simulink model "sampleModel20"  (R2021a)
settings: Solver=VariableStepAuto  StartTime=0.0  StopTime=10.0  RelTol=1e-3
undefined symbols (not defined in the file): DiscIntNeverNeededParam, magnitude, Newton, Raphson
libraries: simulink x274, pid_lib x17
(part 14 of 16)

== system sampleModel20/cfblk90/cfblk9/cfblk9/cfblk5 ==
  cfblk1 : Inport
  cfblk8 : Inport  Port=2
  cfblk10 : Delay  SampleTime=1
  cfblk3 : DiscreteFir  SampleTime=1
  cfblk4 : Sin  TimeSource=Use external signal  SampleTime=0
  cfblk5 : Sum  Inputs=+-
  cfblk6 : ComplexToRealImag
  cfblk7 : MinMax  Inputs=2
  cfblk2 : Outport
  cfblk9 : Outport  Port=2
  wires:
  cfblk8/1 -> cfblk2/1
  cfblk1/1 -> cfblk5/1, cfblk7/2
  cfblk3/1 -> cfblk4/1
  cfblk7/1 -> cfblk6/1
  cfblk5/1 -> cfblk3/1
  cfblk4/1 -> cfblk9/1
  cfblk6/1 -> cfblk5/2
  cfblk6/2 -> cfblk10/1
  cfblk10/1 -> cfblk7/1

== system sampleModel20/cfblk90/cfblk9/cfblk9/cfblk6 ==
  cfblk1 : Inport
  cfblk5 : Inport  Port=2
  cfblk6 : Inport  Port=3
  cfblk7 : Inport  Port=4
  cfblk8 : Inport  Port=5
  cfblk9 : Inport  Port=6
  cfblk10 : Inport  Port=7
  cfblk3 : Reshape
  cfblk4 : Product
  cfblk2 : Outport
  wires:
  cfblk10/1 -> cfblk2/1
  cfblk5/1 -> cfblk4/1
  cfblk1/1 -> cfblk4/2
  cfblk4/1 -> cfblk3/1

== system sampleModel20/cfblk90/cfblk9/cfblk9/cfblk7 ==
  cfblk1 : Inport
  cfblk7 : Inport  Port=2
  cfblk3 : simulink/Math Operations/Slider Gain  gain=1  low=0  high=2
  cfblk4 : Sum  Inputs=+-
  cfblk5 : Product
  cfblk6 : Bias  Bias=[368152443.694758]
  cfblk8 : Delay  SampleTime=1
  cfblk2 : Outport
  wires:
  cfblk3/1 -> cfblk2/1
  cfblk7/1 -> cfblk4/2
  cfblk1/1 -> cfblk3/1
  cfblk4/1 -> cfblk6/1, cfblk5/2
  cfblk6/1 -> cfblk5/1
  cfblk5/1 -> cfblk8/1
  cfblk8/1 -> cfblk4/1

== system sampleModel20/cfblk90/cfblk9/cfblk9/cfblk8 ==
  cfblk1 : Inport
  cfblk6 : Inport  Port=2
  cfblk7 : Inport  Port=3
  cfblk8 : Inport  Port=4
  cfblk9 : Inport  Port=5
  cfblk10 : Inport  Port=6
  cfblk3 : DiscreteTransferFcn  SampleTime=1
  cfblk4 : Product  Inputs=*
  cfblk5 : Reshape
  cfblk2 : Outport
  cfblk11 : Outport  Port=2
  wires:
  cfblk5/1 -> cfblk11/1
  cfblk9/1 -> cfblk5/1
  cfblk10/1 -> cfblk3/1
  cfblk8/1 -> cfblk2/1
  cfblk6/1 -> cfblk4/1

== system sampleModel20/cfblk90/cfblk9/cfblk9/cfblk9 ==
  cfblk1 : Inport
  cfblk10 : Inport  Port=2
  cfblk11 : Inport  Port=3
  cfblk12 : Inport  Port=4
  cfblk13 : Inport  Port=5
  cfblk14 : Inport  Port=6
  cfblk15 : Inport  Port=7
  cfblk17 : Delay  SampleTime=1
  cfblk3 : PermuteDimensions
  cfblk4 : Rounding
  cfblk5 : Product
  cfblk6 : UnaryMinus
  cfblk7 : Signum
  cfblk8 : simulink/Math Operations/Slider Gain  gain=1  low=0  high=2
  cfblk9 : Signum
  cfblk2 : Outport
  cfblk16 : Outport  Port=2
  wires:
  cfblk4/1 -> cfblk3/1
  cfblk7/1 -> cfblk16/1
  cfblk11/1 -> cfblk7/1
  cfblk15/1 -> cfblk6/1
  cfblk10/1 -> cfblk2/1
  cfblk6/1 -> cfblk4/1
  cfblk5/1 -> cfblk8/1
  cfblk1/1 -> cfblk9/1
  cfblk9/1 -> cfblk5/2
  cfblk8/1 -> cfblk17/1
  cfblk17/1 -> cfblk5/1

== system sampleModel20/cfblk91/cfblk5/cfblk10/cfblk10 ==
  cfblk1 : Inport
  cfblk5 : Inport  Port=2
  cfblk6 : Inport  Port=3
  cfblk7 : Inport  Port=4
  cfblk8 : Inport  Port=5
  cfblk9 : Inport  Port=6
  cfblk3 : Sum  Inputs=+-
  cfblk4 : Sum  Inputs=|++
  cfblk2 : Outport
  cfblk10 : Outport  Port=2
  wires:
  cfblk4/1 -> cfblk3/1
  cfblk8/1 -> cfblk2/1
  cfblk7/1 -> cfblk3/2
  cfblk6/1 -> cfblk10/1
  cfblk5/1 -> cfblk4/1
  cfblk1/1 -> cfblk4/2

== system sampleModel20/cfblk91/cfblk5/cfblk10/cfblk11 ==
  cfblk1 : Inport
  cfblk8 : Inport  Port=2
  cfblk9 : Inport  Port=3
  cfblk10 : Inport  Port=4
  cfblk11 : Inport  Port=5
  cfblk12 : Inport  Port=6
  cfblk13 : Inport  Port=7
  cfblk3 : Sqrt  SaturateOnIntegerOverflow=on
  cfblk4 : Sin  TimeSource=Use external signal  SampleTime=0
  cfblk5 : MinMax  Function=max  Inputs=3
  cfblk6 : Squeeze
  cfblk7 : Math  Operator=log10  SaturateOnIntegerOverflow=on
  cfblk2 : Outport
  cfblk14 : Outport  Port=2
  cfblk15 : Outport  Port=3
  wires:
  cfblk11/1 -> cfblk6/1
  cfblk5/1 -> cfblk4/1
  cfblk7/1 -> cfblk15/1
  cfblk1/1 -> cfblk14/1
  cfblk9/1 -> cfblk3/1
  cfblk6/1 -> cfblk2/1
  cfblk8/1 -> cfblk5/1
  cfblk3/1 -> cfblk5/2
  cfblk12/1 -> cfblk7/1
  cfblk13/1 -> cfblk5/3

== system sampleModel20/cfblk91/cfblk5/cfblk10/cfblk12 ==
  cfblk1 : Inport
  cfblk7 : Inport  Port=2
  cfblk8 : Inport  Port=3
  cfblk9 : Inport  Port=4
  cfblk10 : Inport  Port=5
  cfblk11 : Inport  Port=6
  cfblk3 : Sqrt  SaturateOnIntegerOverflow=on
  cfblk4 : Sin  TimeSource=Use external signal  SampleTime=0
  cfblk5 : DotProduct  InputSameDT=on  OutDataTypeStr=Inherit: Inherit via internal rule
  cfblk6 : Polyval  Coefs=[ +2.081618890e-019, -1.441693666e-014, +4.719686976e-010, -8.536869453e-006, +1.621573104e-001, -8.087801117e+001 ]
  cfblk2 : Outport
  cfblk12 : Outport  Port=2
  wires:
  cfblk9/1 -> cfblk5/1
  cfblk11/1 -> cfblk6/1
  cfblk1/1 -> cfblk2/1
  cfblk8/1 -> cfblk4/1
  cfblk5/1 -> cfblk12/1
  cfblk6/1 -> cfblk5/2
  cfblk10/1 -> cfblk3/1

== system sampleModel20/cfblk91/cfblk5/cfblk10/cfblk13 ==
  cfblk1 : Inport
  cfblk5 : Inport  Port=2
  cfblk6 : Inport  Port=3
  cfblk7 : Inport  Port=4
  cfblk3 : Reshape
  cfblk4 : Sin  TimeSource=Use external signal  SampleTime=0
  cfblk2 : Outport
  cfblk8 : Outport  Port=2
  cfblk9 : Outport  Port=3
  wires:
  cfblk6/1 -> cfblk2/1
  cfblk4/1 -> cfblk9/1
  cfblk5/1 -> cfblk4/1
  cfblk1/1 -> cfblk8/1
  cfblk7/1 -> cfblk3/1

== system sampleModel20/cfblk91/cfblk5/cfblk4/cfblk4 ==
  cfblk1 : Inport
  cfblk13 : Inport  Port=2
  cfblk14 : Inport  Port=3
  cfblk10 : Sum  Inputs=|++
  cfblk11 : Polyval  Coefs=[ +2.081618890e-019, -1.441693666e-014, +4.719686976e-010, -8.536869453e-006, +1.621573104e-001, -8.087801117e+001 ]
  cfblk12 : Assignment  DiagnosticForDimensions=Warning  IndexOptions=Index vector (dialog)  Indices=1  OutputSizes=1
  cfblk15 : Delay  SampleTime=1
  cfblk16 : Delay  SampleTime=1
  cfblk3 : Rounding
  cfblk4 : ComplexToRealImag
  cfblk5 : Abs
  cfblk6 : Sum  Inputs=|++
  cfblk7 : ComplexToMagnitudeAngle
  cfblk8 : simulink/Math Operations/MinMax Running Resettable  Function=min  vinit=0.0
  cfblk9 : Product  Inputs=**
  cfblk2 : Outport
  wires:
  cfblk14/1 -> cfblk12/1
  cfblk1/1 -> cfblk4/1, cfblk5/1
  cfblk4/1 -> cfblk2/1
  cfblk13/1 -> cfblk10/1
  cfblk6/1 -> cfblk7/1
  cfblk9/1 -> cfblk3/1
  cfblk11/1 -> cfblk6/2
  cfblk12/1 -> cfblk9/1
  cfblk7/2 -> cfblk8/2
  cfblk8/1 -> cfblk12/2
  cfblk10/1 -> cfblk9/2
  cfblk5/1 -> cfblk10/2
  cfblk4/2 -> cfblk11/1
  cfblk7/1 -> cfblk15/1
  cfblk15/1 -> cfblk6/1
  cfblk3/1 -> cfblk16/1
  cfblk16/1 -> cfblk8/1

== system sampleModel20/cfblk91/cfblk5/cfblk4/cfblk5 ==
  cfblk1 : Inport
  cfblk7 : Inport  Port=2
  cfblk8 : Inport  Port=3
  cfblk9 : Inport  Port=4
  cfblk12 : Delay  SampleTime=1
  cfblk3 : ComplexToMagnitudeAngle
  cfblk4 : PermuteDimensions
  cfblk5 : Sin  TimeSource=Use external signal  SampleTime=0
  cfblk6 : Product  Inputs=**
  cfblk2 : Outport
  cfblk10 : Outport  Port=2
  cfblk11 : Outport  Port=3
  wires:
  cfblk3/1 -> cfblk11/1
  cfblk8/1 -> cfblk4/1
  cfblk9/1 -> cfblk10/1
  cfblk1/1 -> cfblk2/1
  cfblk5/1 -> cfblk6/1
  cfblk3/2 -> cfblk5/1
  cfblk7/1 -> cfblk6/2
  cfblk6/1 -> cfblk12/1
  cfblk12/1 -> cfblk3/1

== system sampleModel20/cfblk91/cfblk5/cfblk5/cfblk8 ==
  cfblk1 : Inport
  cfblk10 : Inport  Port=2
  cfblk11 : Inport  Port=3
  cfblk12 : Inport  Port=4
  cfblk13 : Inport  Port=5
  cfblk14 : Inport  Port=6
  cfblk15 : Inport  Port=7
  cfblk16 : Inport  Port=8
  cfblk17 : Inport  Port=9
  cfblk3 : PermuteDimensions
  cfblk4 : Reshape
  cfblk5 : Abs
  cfblk6 : Assignment  DiagnosticForDimensions=Warning  IndexOptions=Index vector (dialog)  Indices=1  OutputSizes=1
  cfblk7 : MinMax  Inputs=2
  cfblk8 : simulink/Math Operations/MinMax Running Resettable  Function=min  vinit=0.0
  cfblk9 : Product  Inputs=**
  cfblk2 : Outport
  wires:
  cfblk6/1 -> cfblk4/1
  cfblk1/1 -> cfblk5/1
  cfblk10/1 -> cfblk6/1
  cfblk17/1 -> cfblk7/1
  cfblk13/1 -> cfblk3/1
  cfblk11/1 -> cfblk9/1
  cfblk14/1 -> cfblk8/1
  cfblk3/1 -> cfblk2/1
  cfblk12/1 -> cfblk9/2
  cfblk8/1 -> cfblk7/2
  cfblk16/1 -> cfblk6/2
  cfblk15/1 -> cfblk8/2

== system sampleModel20/cfblk91/cfblk5/cfblk5/cfblk9 ==
  cfblk1 : Inport
  cfblk5 : Inport  Port=2
  cfblk6 : Inport  Port=3
  cfblk7 : Inport  Port=4
  cfblk3 : Sum  Inputs=+-
  cfblk4 : Sum  Inputs=|++
  cfblk2 : Outport
  wires:
  cfblk3/1 -> cfblk4/1
  cfblk1/1 -> cfblk2/1
  cfblk5/1 -> cfblk4/2
  cfblk7/1 -> cfblk3/1
  cfblk6/1 -> cfblk3/2

== system sampleModel20/cfblk91/cfblk5/cfblk6/cfblk5 ==
  cfblk1 : Inport
  cfblk9 : Inport  Port=2
  cfblk10 : Inport  Port=3
  cfblk11 : Inport  Port=4
  cfblk12 : Inport  Port=5
  cfblk13 : Inport  Port=6
  cfblk14 : Inport  Port=7
  cfblk3 : Sqrt  SaturateOnIntegerOverflow=on
  cfblk4 : Reshape
  cfblk5 : MinMax  Function=max
  cfblk6 : PermuteDimensions
  cfblk7 : ComplexToMagnitudeAngle
  cfblk8 : simulink/Math Operations/Slider Gain  gain=1  low=0  high=2
  cfblk2 : Outport
  wires:
  cfblk8/1 -> cfblk2/1
  cfblk4/1 -> cfblk6/1
  cfblk1/1 -> cfblk5/1
  cfblk12/1 -> cfblk7/1
  cfblk3/1 -> cfblk8/1
  cfblk11/1 -> cfblk4/1
  cfblk9/1 -> cfblk3/1

== system sampleModel20/cfblk91/cfblk5/cfblk7/cfblk5 ==
  cfblk1 : Inport
  cfblk6 : Inport  Port=2
  cfblk7 : Inport  Port=3
  cfblk8 : Inport  Port=4
  cfblk9 : Inport  Port=5
  cfblk10 : Inport  Port=6
  cfblk11 : Inport  Port=7
  cfblk16 : Delay  SampleTime=1
  cfblk3 : Assignment  DiagnosticForDimensions=Warning  IndexOptions=Index vector (dialog)  Indices=1  OutputSizes=1
  cfblk4 : MinMax  Function=max
  cfblk5 : ComplexToMagnitudeAngle
  cfblk2 : Outport
  cfblk12 : Outport  Port=2
  cfblk13 : Outport  Port=3
  cfblk14 : Outport  Port=4
  cfblk15 : Outport  Port=5
  wires:
  cfblk11/1 -> cfblk13/1
  cfblk1/1 -> cfblk2/1
  cfblk3/1 -> cfblk5/1
  cfblk4/1 -> cfblk3/1
  cfblk6/1 -> cfblk4/1
  cfblk9/1 -> cfblk14/1
  cfblk7/1 -> cfblk12/1
  cfblk10/1 -> cfblk15/1
  cfblk5/1 -> cfblk16/1
  cfblk16/1 -> cfblk3/2

== system sampleModel20/cfblk91/cfblk5/cfblk7/cfblk6 ==
  cfblk1 : Inport
  cfblk8 : Inport  Port=2
  cfblk11 : Delay  SampleTime=1
  cfblk3 : Assignment  DiagnosticForDimensions=Warning  IndexOptions=Index vector (dialog)  Indices=1  OutputSizes=1
  cfblk4 : simulink/Math Operations/Slider Gain  gain=1  low=0  high=2
  cfblk5 : Math  Operator=rem  SaturateOnIntegerOverflow=on
  cfblk6 : ComplexToRealImag
  cfblk7 : Constant  Value=[-196577758.764814]  SampleTime=1
  cfblk2 : Outport
  cfblk9 : Outport  Port=2
  cfblk10 : Outport  Port=3
  wires:
  cfblk5/1 -> cfblk4/1
  cfblk8/1 -> cfblk2/1, cfblk3/2
  cfblk1/1 -> cfblk5/1
  cfblk4/1 -> cfblk10/1
  cfblk3/1 -> cfblk6/1
  cfblk7/1 -> cfblk5/2
  cfblk6/1 -> cfblk9/1
  cfblk6/2 -> cfblk11/1
  cfblk11/1 -> cfblk3/1

== system sampleModel20/cfblk91/cfblk5/cfblk7/cfblk7 ==
  cfblk1 : Inport
  cfblk8 : Inport  Port=2
  cfblk9 : Inport  Port=3
  cfblk10 : Inport  Port=4
  cfblk11 : Inport  Port=5
  cfblk12 : Inport  Port=6
  cfblk15 : Delay  SampleTime=1
  cfblk16 : Delay  SampleTime=1
  cfblk3 : Sum  Inputs=|++
  cfblk4 : ComplexToMagnitudeAngle
  cfblk5 : Sum  Inputs=+-
  cfblk6 : Signum
  cfblk7 : Product
  cfblk2 : Outport
  cfblk13 : Outport  Port=2
  cfblk14 : Outport  Port=3
  wires:
  cfblk9/1 -> cfblk5/1
  cfblk12/1 -> cfblk5/2
  cfblk1/1 -> cfblk6/1
  cfblk6/1 -> cfblk2/1
  cfblk11/1 -> cfblk13/1
  cfblk5/1 -> cfblk7/1
  cfblk3/1 -> cfblk4/1
  cfblk8/1 -> cfblk14/1
  cfblk4/2 -> cfblk7/2
  cfblk4/1 -> cfblk15/1
  cfblk15/1 -> cfblk3/2
  cfblk7/1 -> cfblk16/1
  cfblk16/1 -> cfblk3/1

== system sampleModel20/cfblk91/cfblk5/cfblk7/cfblk8 ==
  cfblk1 : Inport
  cfblk5 : Inport  Port=2
  cfblk6 : Inport  Port=3
  cfblk7 : Inport  Port=4
  cfblk3 : Product
  cfblk4 : Bias  Bias=[403133249.538603]
  cfblk2 : Outport
  wires:
  cfblk3/1 -> cfblk4/1
  cfblk4/1 -> cfblk2/1
  cfblk7/1 -> cfblk3/1
  cfblk5/1 -> cfblk3/2

== system sampleModel20/cfblk91/cfblk5/cfblk8/cfblk5 ==
  cfblk1 : Inport
  cfblk6 : Inport  Port=2
  cfblk7 : Inport  Port=3
  cfblk8 : Inport  Port=4
  cfblk9 : Inport  Port=5
  cfblk10 : Inport  Port=6
  cfblk3 : Gain  Gain=[791787314.967177]
  cfblk4 : Gain  Gain=[648519034.471497]
  cfblk5 : Abs
  cfblk2 : Outport
  cfblk11 : Outport  Port=2
  cfblk12 : Outport  Port=3
  cfblk13 : Outport  Port=4
  cfblk14 : Outport  Port=5
  wires:
  cfblk6/1 -> cfblk13/1
  cfblk10/1 -> cfblk2/1
  cfblk3/1 -> cfblk4/1
  cfblk1/1 -> cfblk12/1
  cfblk7/1 -> cfblk14/1
  cfblk8/1 -> cfblk5/1
  cfblk5/1 -> cfblk11/1
  cfblk9/1 -> cfblk3/1

== system sampleModel20/cfblk91/cfblk5/cfblk8/cfblk6 ==
  cfblk1 : Inport
  cfblk4 : Inport  Port=2
  cfblk5 : Inport  Port=3
  cfblk6 : Inport  Port=4
  cfblk7 : Inport  Port=5
  cfblk3 : Sum  Inputs=+
  cfblk2 : Outport
  wires:
  cfblk3/1 -> cfblk2/1
  cfblk1/1 -> cfblk3/1

== system sampleModel20/cfblk91/cfblk5/cfblk8/cfblk7 ==
  cfblk1 : Inport
  cfblk7 : Inport  Port=2
  cfblk8 : Inport  Port=3
  cfblk9 : Inport  Port=4
  cfblk10 : Inport  Port=5
  cfblk11 : Inport  Port=6
  cfblk12 : Inport  Port=7
  cfblk13 : Inport  Port=8
  cfblk15 : Delay  SampleTime=1
  cfblk3 : DiscreteIntegrator  ICPrevOutput=DiscIntNeverNeededParam  ICPrevScaledInput=DiscIntNeverNeededParam
  cfblk4 : DotProduct  InputSameDT=on  OutDataTypeStr=Inherit: Inherit via internal rule
  cfblk5 : Sum  Inputs=+-
  cfblk6 : Assignment  DiagnosticForDimensions=Warning  IndexOptions=Index vector (dialog)  Indices=1  OutputSizes=1
  cfblk2 : Outport
  cfblk14 : Outport  Port=2
  wires:
  cfblk12/1 -> cfblk2/1
  cfblk4/1 -> cfblk6/1
  cfblk8/1 -> cfblk5/1
  cfblk7/1 -> cfblk14/1
  cfblk10/1 -> cfblk5/2
  cfblk1/1 -> cfblk4/2
  cfblk11/1 -> cfblk3/1
  cfblk3/1 -> cfblk6/2
  cfblk6/1 -> cfblk15/1
  cfblk15/1 -> cfblk4/1

== system sampleModel20/cfblk91/cfblk5/cfblk8/cfblk8 ==
  cfblk1 : Inport
  cfblk10 : Inport  Port=2
  cfblk14 : Delay  SampleTime=1
  cfblk3 : MinMax  Function=max
  cfblk4 : Sum  Inputs=+
  cfblk5 : Product
  cfblk6 : ComplexToMagnitudeAngle
  cfblk7 : simulink/Math Operations/MinMax Running Resettable  Function=min  vinit=0.0
  cfblk8 : Signum
  cfblk9 : Sin  TimeSource=Use external signal  SampleTime=0
  cfblk2 : Outport
  cfblk11 : Outport  Port=2
  cfblk12 : Outport  Port=3
  cfblk13 : Outport  Port=4
  wires:
  cfblk7/1 -> cfblk12/1, cfblk9/1
  cfblk3/1 -> cfblk4/1
  cfblk5/1 -> cfblk7/1, cfblk3/1
  cfblk4/1 -> cfblk2/1
  cfblk10/1 -> cfblk8/1, cfblk7/2
  cfblk9/1 -> cfblk6/1
  cfblk1/1 -> cfblk11/1
  cfblk8/1 -> cfblk5/2
  cfblk6/2 -> cfblk13/1
  cfblk6/1 -> cfblk14/1
  cfblk14/1 -> cfblk5/1

== system sampleModel20/cfblk91/cfblk5/cfblk9/cfblk10 ==
  cfblk1 : Inport
  cfblk6 : Inport  Port=2
  cfblk7 : Inport  Port=3
  cfblk3 : UnaryMinus
  cfblk4 : Signum
  cfblk5 : Constant  Value=[-814383942.447374]  SampleTime=1
  cfblk2 : Outport
  cfblk8 : Outport  Port=2
  wires:
  cfblk5/1 -> cfblk2/1
  cfblk1/1 -> cfblk4/1
  cfblk6/1 -> cfblk3/1
  cfblk7/1 -> cfblk8/1

== system sampleModel20/cfblk91/cfblk5/cfblk9/cfblk11 ==
  cfblk1 : Inport
  cfblk8 : Inport  Port=2
  cfblk9 : Inport  Port=3
  cfblk10 : Inport  Port=4
  cfblk11 : Inport  Port=5
  cfblk12 : Inport  Port=6
  cfblk13 : Inport  Port=7
  cfblk14 : Inport  Port=8
  cfblk15 : Inport  Port=9
  cfblk3 : UnaryMinus
  cfblk4 : Sum  Inputs=--
  cfblk5 : Sum  Inputs=+
  cfblk6 : simulink/Math Operations/Slider Gain  gain=1  low=0  high=2
  cfblk7 : Sum  Inputs=+
  cfblk2 : Outport
  wires:
  cfblk15/1 -> cfblk6/1
  cfblk9/1 -> cfblk4/1
  cfblk5/1 -> cfblk4/2
  cfblk13/1 -> cfblk7/1
  cfblk8/1 -> cfblk2/1
  cfblk6/1 -> cfblk5/1
  cfblk11/1 -> cfblk3/1

== system sampleModel20/cfblk91/cfblk5/cfblk9/cfblk12 ==
  cfblk1 : Inport
  cfblk9 : Inport  Port=2
  cfblk10 : Inport  Port=3
  cfblk11 : Inport  Port=4
  cfblk12 : Inport  Port=5
  cfblk13 : Inport  Port=6
  cfblk14 : Inport  Port=7
  cfblk3 : simulink/Discrete/Transfer Fcn First Order  PoleZ=0.95  ICPrevOutput=0.0  DoSatur=off
  cfblk4 : simulink/Math Operations/MinMax Running Resettable  Function=min  vinit=0.0
  cfblk5 : Reshape
  cfblk6 : ComplexToRealImag
  cfblk7 : Sqrt  SaturateOnIntegerOverflow=on
  cfblk8 : Product  Inputs=**
  cfblk2 : Outport
  wires:
  cfblk5/1 -> cfblk4/1
  cfblk6/1 -> cfblk5/1
  cfblk7/1 -> cfblk4/2
  cfblk12/1 -> cfblk6/1
  cfblk13/1 -> cfblk7/1
  cfblk11/1 -> cfblk8/1
  cfblk10/1 -> cfblk8/2
  cfblk6/2 -> cfblk3/1
  cfblk14/1 -> cfblk2/1

== system sampleModel20/cfblk91/cfblk5/cfblk9/cfblk9 ==
  cfblk1 : Inport
  cfblk9 : Inport  Port=2
  cfblk12 : Delay  SampleTime=1
  cfblk13 : Delay  SampleTime=1
  cfblk3 : UnaryMinus
  cfblk4 : Product  Inputs=*
  cfblk5 : Sum  Inputs=-+
  cfblk6 : Gain  Gain=[789098351.515024]
  cfblk7 : simulink/Math Operations/MinMax Running Resettable  Function=min  vinit=0.0
  cfblk8 : MinMax  Function=max  Inputs=2
  cfblk2 : Outport
  cfblk10 : Outport  Port=2
  cfblk11 : Outport  Port=3
  wires:
  cfblk8/1 -> cfblk4/1, cfblk13/1
  cfblk7/1 -> cfblk8/1
  cfblk4/1 -> cfblk5/1, cfblk11/1
  cfblk1/1 -> cfblk6/1
  cfblk3/1 -> cfblk5/2
  cfblk9/1 -> cfblk3/1
  cfblk6/1 -> cfblk10/1, cfblk2/1, cfblk7/1
  cfblk5/1 -> cfblk12/1
  cfblk12/1 -> cfblk8/2
  cfblk13/1 -> cfblk7/2

== system sampleModel20/cfblk91/cfblk7/cfblk4/cfblk4 ==
  cfblk1 : Inport
  cfblk5 : Inport  Port=2
  cfblk6 : Inport  Port=3
  cfblk7 : Inport  Port=4
  cfblk8 : Inport  Port=5
  cfblk9 : Inport  Port=6
  cfblk10 : Inport  Port=7
  cfblk11 : Inport  Port=8
  cfblk12 : Inport  Port=9
  cfblk13 : Inport  Port=10
  cfblk3 : Squeeze
  cfblk4 : Assignment  DiagnosticForDimensions=Warning  IndexOptions=Index vector (dialog)  Indices=1  OutputSizes=1
  cfblk2 : Outport
  cfblk14 : Outport  Port=2
  wires:
  cfblk5/1 -> cfblk3/1
  cfblk1/1 -> cfblk2/1
  cfblk9/1 -> cfblk4/1
  cfblk10/1 -> cfblk14/1
  cfblk7/1 -> cfblk4/2

== system sampleModel20/cfblk91/cfblk7/cfblk5/cfblk4 ==
  cfblk1 : Inport
  cfblk5 : Inport  Port=2
  cfblk6 : Inport  Port=3
  cfblk3 : Rounding
  cfblk4 : Squeeze
  cfblk2 : Outport
  cfblk7 : Outport  Port=2
  wires:
  cfblk3/1 -> cfblk2/1
  cfblk4/1 -> cfblk7/1
  cfblk1/1 -> cfblk3/1
  cfblk6/1 -> cfblk4/1

== system sampleModel20/cfblk91/cfblk7/cfblk5/cfblk5 ==
  cfblk1 : Inport
  cfblk9 : Inport  Port=2
  cfblk10 : Inport  Port=3
  cfblk11 : Inport  Port=4
  cfblk12 : Inport  Port=5
  cfblk13 : Inport  Port=6
  cfblk14 : Inport  Port=7
  cfblk3 : Product
  cfblk4 : Product  Inputs=**
  cfblk5 : Sqrt  SaturateOnIntegerOverflow=on
  cfblk6 : Product  Inputs=*
  cfblk7 : Product  Inputs=*
  cfblk8 : Rounding
  cfblk2 : Outport
  cfblk15 : Outport  Port=2
  wires:
  cfblk5/1 -> cfblk15/1
  cfblk12/1 -> cfblk6/1
  cfblk13/1 -> cfblk7/1
  cfblk9/1 -> cfblk4/1
  cfblk4/1 -> cfblk8/1
  cfblk14/1 -> cfblk2/1
  cfblk6/1 -> cfblk4/2
  cfblk11/1 -> cfblk3/1
  cfblk7/1 -> cfblk3/2
  cfblk3/1 -> cfblk5/1

== system sampleModel20/cfblk91/cfblk8/cfblk6/cfblk3 ==
  cfblk1 : Inport
  cfblk6 : Inport  Port=2
  cfblk7 : Inport  Port=3
  cfblk3 : Sum
  cfblk4 : Math  SaturateOnIntegerOverflow=on
  cfblk5 : MinMax  Function=max  Inputs=2
  cfblk8 : Delay  SampleTime=1
  cfblk2 : Outport
  wires:
  cfblk1/1 -> cfblk3/1
  cfblk7/1 -> cfblk2/1
  cfblk3/1 -> cfblk4/1
  cfblk4/1 -> cfblk5/1
  cfblk6/1 -> cfblk5/2
  cfblk5/1 -> cfblk8/1
  cfblk8/1 -> cfblk3/2

== system sampleModel20/cfblk91/cfblk8/cfblk6/cfblk4 ==
  cfblk1 : Inport
  cfblk10 : Inport  Port=2
  cfblk11 : Inport  Port=3
  cfblk12 : Inport  Port=4
  cfblk13 : Inport  Port=5
  cfblk14 : Inport  Port=6
  cfblk3 : Squeeze
  cfblk4 : Product  Inputs=*
  cfblk5 : Product  Inputs=**
  cfblk6 : PermuteDimensions
  cfblk7 : Abs
  cfblk8 : Assignment  DiagnosticForDimensions=Warning  IndexOptions=Index vector (dialog)  Indices=1  OutputSizes=1
  cfblk9 : MinMax
  cfblk2 : Outport
  cfblk15 : Outport  Port=2
  wires:
  cfblk9/1 -> cfblk3/1
  cfblk3/1 -> cfblk4/1
  cfblk4/1 -> cfblk7/1
  cfblk12/1 -> cfblk9/1
  cfblk13/1 -> cfblk15/1
  cfblk5/1 -> cfblk8/1
  cfblk14/1 -> cfblk5/1
  cfblk1/1 -> cfblk2/1
  cfblk8/1 -> cfblk6/1
  cfblk11/1 -> cfblk8/2
  cfblk10/1 -> cfblk5/2

== system sampleModel20/cfblk91/cfblk8/cfblk6/cfblk5 ==
  cfblk1 : Inport
  cfblk8 : Inport  Port=2
  cfblk9 : Inport  Port=3
  cfblk3 : DiscreteZeroPole  Poles=[0 0.5]  Gain=1
  cfblk4 : Polyval  Coefs=[ +2.081618890e-019, -1.441693666e-014, +4.719686976e-010, -8.536869453e-006, +1.621573104e-001, -8.087801117e+001 ]
  cfblk5 : Sum  Inputs=|++
  cfblk6 : Product  Inputs=*
  cfblk7 : ComplexToMagnitudeAngle
  cfblk2 : Outport
  wires:
  cfblk4/1 -> cfblk5/1
  cfblk9/1 -> cfblk4/1
  cfblk1/1 -> cfblk6/1
  cfblk6/1 -> cfblk3/1
  cfblk5/1 -> cfblk7/1
  cfblk3/1 -> cfblk2/1
  cfblk8/1 -> cfblk5/2

== system sampleModel20/cfblk91/cfblk8/cfblk7/cfblk7 ==
  cfblk1 : Inport
  cfblk5 : Inport  Port=2
  cfblk6 : Inport  Port=3
  cfblk7 : Inport  Port=4
  cfblk8 : Inport  Port=5
  cfblk9 : Inport  Port=6
  cfblk3 : DiscreteZeroPole  Poles=[0 0.5]  Gain=1
  cfblk4 : Rounding
  cfblk2 : Outport
  wires:
  cfblk1/1 -> cfblk4/1
  cfblk7/1 -> cfblk3/1
  cfblk6/1 -> cfblk2/1

== system sampleModel20/cfblk91/cfblk8/cfblk7/cfblk8 ==
  cfblk1 : Inport
  cfblk5 : Inport  Port=2
  cfblk6 : Inport  Port=3
  cfblk7 : Inport  Port=4
  cfblk8 : Inport  Port=5
  cfblk9 : Inport  Port=6
  cfblk10 : Inport  Port=7
  cfblk11 : Inport  Port=8
  cfblk3 : Sqrt  SaturateOnIntegerOverflow=on
  cfblk4 : UnaryMinus
  cfblk2 : Outport
  cfblk12 : Outport  Port=2
  wires:
  cfblk6/1 -> cfblk2/1
  cfblk5/1 -> cfblk12/1
  cfblk11/1 -> cfblk4/1
  cfblk4/1 -> cfblk3/1

== system sampleModel20/cfblk91/cfblk8/cfblk8/cfblk4 ==
  cfblk1 : Inport
  cfblk8 : Inport  Port=2
  cfblk10 : Delay  SampleTime=1
  cfblk3 : Sum  Inputs=|++
  cfblk4 : Rounding
  cfblk5 : Sum  Inputs=--
  cfblk6 : Sin  TimeSource=Use external signal  SampleTime=0
  cfblk7 : Sum  Inputs=|++
  cfblk2 : Outport
  cfblk9 : Outport  Port=2
  wires:
  cfblk6/1 -> cfblk5/1
  cfblk1/1 -> cfblk7/1, cfblk5/2
  cfblk5/1 -> cfblk9/1
  cfblk7/1 -> cfblk6/1, cfblk3/2
  cfblk8/1 -> cfblk4/1, cfblk3/1
  cfblk4/1 -> cfblk2/1
  cfblk3/1 -> cfblk10/1
  cfblk10/1 -> cfblk7/2

== system sampleModel20/cfblk93/cfblk6/cfblk9/cfblk11 ==
  cfblk1 : Inport
  cfblk4 : Inport  Port=2
  cfblk5 : Inport  Port=3
  cfblk6 : Inport  Port=4
  cfblk3 : Product  Inputs=**
  cfblk2 : Outport
  cfblk7 : Outport  Port=2
  wires:
  cfblk4/1 -> cfblk3/1
  cfblk3/1 -> cfblk2/1
  cfblk5/1 -> cfblk3/2
  cfblk6/1 -> cfblk7/1

== system sampleModel20/cfblk93/cfblk6/cfblk9/cfblk12 ==
  cfblk1 : Inport
  cfblk11 : Inport  Port=2
  cfblk12 : Inport  Port=3
  cfblk13 : Inport  Port=4
  cfblk14 : Inport  Port=5
  cfblk15 : Inport  Port=6
  cfblk16 : Inport  Port=7
  cfblk10 : Sum  Inputs=+
  cfblk3 : UnitDelay  HasFrameUpgradeWarning=on
  cfblk4 : Bias  Bias=[-369034193.627380]
  cfblk5 : Abs
  cfblk6 : Sin  TimeSource=Use external signal  SampleTime=0
  cfblk7 : Trigonometry
  cfblk8 : MinMax  Function=max
  cfblk9 : ComplexToRealImag
  cfblk2 : Outport
  wires:
  cfblk11/1 -> cfblk7/1
  cfblk5/1 -> cfblk9/1
  cfblk13/1 -> cfblk5/1
  cfblk15/1 -> cfblk8/1
  cfblk8/1 -> cfblk3/1
  cfblk1/1 -> cfblk10/1
  cfblk3/1 -> cfblk2/1
  cfblk10/1 -> cfblk6/1
  cfblk16/1 -> cfblk4/1

== system sampleModel20/cfblk93/cfblk7/cfblk10/cfblk4 ==
  cfblk1 : Inport
  cfblk9 : Inport  Port=2
  cfblk10 : Inport  Port=3
  cfblk11 : Inport  Port=4
  cfblk12 : Inport  Port=5
  cfblk13 : Inport  Port=6
  cfblk14 : Inport  Port=7
  cfblk15 : Inport  Port=8
  cfblk18 : Delay  SampleTime=1
  cfblk3 : Sin  TimeSource=Use external signal  SampleTime=0
  cfblk4 : DotProduct  InputSameDT=on  OutDataTypeStr=Inherit: Inherit via internal rule
  cfblk5 : Sum  Inputs=|++
  cfblk6 : Polyval  Coefs=[ +2.081618890e-019, -1.441693666e-014, +4.719686976e-010, -8.536869453e-006, +1.621573104e-001, -8.087801117e+001 ]
  cfblk7 : Sum  Inputs=|++
  cfblk8 : Gain  Gain=[847959377.972689]
  cfblk2 : Outport
  cfblk16 : Outport  Port=2
  cfblk17 : Outport  Port=3
  wires:
  cfblk14/1 -> cfblk2/1
  cfblk15/1 -> cfblk4/1
  cfblk1/1 -> cfblk6/1
  cfblk13/1 -> cfblk4/2
  cfblk8/1 -> cfblk3/1
  cfblk12/1 -> cfblk5/2
  cfblk6/1 -> cfblk8/1
  cfblk5/1 -> cfblk7/1
  cfblk9/1 -> cfblk16/1
  cfblk10/1 -> cfblk7/2
  cfblk3/1 -> cfblk17/1
  cfblk7/1 -> cfblk18/1
  cfblk18/1 -> cfblk5/1

== system sampleModel20/cfblk93/cfblk7/cfblk10/cfblk5 ==
  cfblk1 : Inport
  cfblk6 : Inport  Port=2
  cfblk7 : Inport  Port=3
  cfblk8 : Inport  Port=4
  cfblk9 : Inport  Port=5
  cfblk10 : Inport  Port=6
  cfblk11 : Inport  Port=7
  cfblk3 : Product  Inputs=**
  cfblk4 : Sum  Inputs=--
  cfblk5 : Trigonometry
  cfblk2 : Outport
  wires:
  cfblk7/1 -> cfblk5/1
  cfblk8/1 -> cfblk4/1
  cfblk1/1 -> cfblk2/1
  cfblk9/1 -> cfblk3/1
  cfblk3/1 -> cfblk4/2
  cfblk10/1 -> cfblk3/2

== system sampleModel20/cfblk94/cfblk10/cfblk6/cfblk5 ==
  cfblk1 : Inport
  cfblk5 : Inport  Port=2
  cfblk6 : Inport  Port=3
  cfblk7 : Inport  Port=4
  cfblk8 : Inport  Port=5
  cfblk3 : Sum  Inputs=+-
  cfblk4 : Sqrt  Operator=rSqrt  AlgorithmType=Newton-Raphson  SaturateOnIntegerOverflow=on
  cfblk2 : Outport
  cfblk9 : Outport  Port=2
  wires:
  cfblk8/1 -> cfblk2/1
  cfblk6/1 -> cfblk3/1
  cfblk4/1 -> cfblk3/2
  cfblk5/1 -> cfblk4/1
  cfblk3/1 -> cfblk9/1

== system sampleModel20/cfblk94/cfblk10/cfblk7/cfblk4 ==
  cfblk1 : Inport
  cfblk7 : Inport  Port=2
  cfblk8 : Inport  Port=3
  cfblk9 : Inport  Port=4
  cfblk10 : Inport  Port=5
  cfblk11 : Inport  Port=6
  cfblk12 : Inport  Port=7
  cfblk13 : Inport  Port=8
  cfblk14 : Inport  Port=9
  cfblk15 : Delay  SampleTime=1
  cfblk3 : Sum  Inputs=|++
  cfblk4 : Gain  Gain=[-773000732.519584]
  cfblk5 : Sqrt  SaturateOnIntegerOverflow=on
  cfblk6 : Sum  Inputs=+
  cfblk2 : Outport
  wires:
  cfblk13/1 -> cfblk5/1
  cfblk12/1 -> cfblk2/1
  cfblk4/1 -> cfblk6/1
  cfblk9/1 -> cfblk3/1
  cfblk11/1 -> cfblk3/2
  cfblk6/1 -> cfblk15/1
  cfblk15/1 -> cfblk4/1

== system sampleModel20/cfblk94/cfblk10/cfblk7/cfblk5 ==
  cfblk1 : Inport
  cfblk11 : Inport  Port=2
  cfblk12 : Inport  Port=3
  cfblk13 : Inport  Port=4
  cfblk14 : Inport  Port=5
  cfblk15 : Inport  Port=6
  cfblk10 : Gain  Gain=[-264021520.597620]
  cfblk3 : Product
  cfblk4 : Reshape
  cfblk5 : simulink/Math Operations/Slider Gain  gain=1  low=0  high=2
  cfblk6 : Polyval  Coefs=[ +2.081618890e-019, -1.441693666e-014, +4.719686976e-010, -8.536869453e-006, +1.621573104e-001, -8.087801117e+001 ]
  cfblk7 : Product  Inputs=*
  cfblk8 : PermuteDimensions
  cfblk9 : Product  Inputs=**
  cfblk2 : Outport
  cfblk16 : Outport  Port=2
  cfblk17 : Outport  Port=3
  wires:
  cfblk11/1 -> cfblk9/1
  cfblk1/1 -> cfblk17/1
  cfblk12/1 -> cfblk6/1
  cfblk4/1 -> cfblk16/1
  cfblk8/1 -> cfblk7/1
  cfblk6/1 -> cfblk5/1
  cfblk15/1 -> cfblk8/1
  cfblk9/1 -> cfblk3/1
  cfblk5/1 -> cfblk9/2
  cfblk14/1 -> cfblk3/2
  cfblk13/1 -> cfblk10/1
  cfblk7/1 -> cfblk2/1
  cfblk3/1 -> cfblk4/1

== system sampleModel20/cfblk94/cfblk10/cfblk7/cfblk6 ==
  cfblk1 : Inport
  cfblk10 : Inport  Port=2
  cfblk11 : Inport  Port=3
  cfblk12 : Inport  Port=4
  cfblk13 : Inport  Port=5
  cfblk15 : Delay  SampleTime=1
  cfblk3 : Sum  Inputs=--
  cfblk4 : Math  Operator=magnitude^2  SaturateOnIntegerOverflow=on
  cfblk5 : Sum  Inputs=+-
  cfblk6 : simulink/Math Operations/Slider Gain  gain=1  low=0  high=2
  cfblk7 : DotProduct  InputSameDT=on  OutDataTypeStr=Inherit: Inherit via internal rule
  cfblk8 : Product
  cfblk9 : Squeeze
  cfblk2 : Outport
  cfblk14 : Outport  Port=2
  wires:
  cfblk11/1 -> cfblk6/1
  cfblk4/1 -> cfblk2/1
  cfblk9/1 -> cfblk8/1
  cfblk8/1 -> cfblk7/1
  cfblk7/1 -> cfblk4/1, cfblk3/2
  cfblk6/1 -> cfblk9/1
  cfblk3/1 -> cfblk5/1
  cfblk12/1 -> cfblk5/2
  cfblk13/1 -> cfblk8/2
  cfblk1/1 -> cfblk7/2
  cfblk10/1 -> cfblk14/1
  cfblk5/1 -> cfblk15/1
  cfblk15/1 -> cfblk3/1

== system sampleModel20/cfblk94/cfblk10/cfblk7/cfblk7 ==
  cfblk1 : Inport
  cfblk10 : Inport  Port=2
  cfblk11 : Inport  Port=3
  cfblk12 : Inport  Port=4
  cfblk13 : Inport  Port=5
  cfblk14 : Inport  Port=6
  cfblk15 : Inport  Port=7
  cfblk16 : Inport  Port=8
  cfblk3 : Signum
  cfblk4 : Bias  Bias=[-910830288.784640]
  cfblk5 : Trigonometry
  cfblk6 : MinMax  Function=max  Inputs=2
  cfblk7 : simulink/Math Operations/MinMax Running Resettable  Function=min  vinit=0.0
  cfblk8 : Constant  Value=[925271336.014879]  SampleTime=1
  cfblk9 : Constant  Value=[-156888013.743022]  SampleTime=1
  cfblk2 : Outport
  cfblk17 : Outport  Port=2
  wires:
  cfblk4/1 -> cfblk17/1
  cfblk10/1 -> cfblk4/1
  cfblk5/1 -> cfblk6/1
  cfblk3/1 -> cfblk5/1
  cfblk8/1 -> cfblk6/2
  cfblk11/1 -> cfblk7/1
  cfblk14/1 -> cfblk7/2
  cfblk16/1 -> cfblk2/1
  cfblk15/1 -> cfblk3/1

== system sampleModel20/cfblk94/cfblk10/cfblk7/cfblk8 ==
  cfblk1 : Inport
  cfblk4 : Inport  Port=2
  cfblk5 : Inport  Port=3
  cfblk6 : Inport  Port=4
  cfblk7 : Inport  Port=5
  cfblk8 : Inport  Port=6
  cfblk9 : Inport  Port=7
  cfblk3 : Sqrt  SaturateOnIntegerOverflow=on
  cfblk2 : Outport
  cfblk10 : Outport  Port=2
  cfblk11 : Outport  Port=3
  wires:
  cfblk8/1 -> cfblk2/1
  cfblk1/1 -> cfblk11/1
  cfblk4/1 -> cfblk3/1
  cfblk7/1 -> cfblk10/1

== system sampleModel20/cfblk94/cfblk10/cfblk7/cfblk9 ==
  cfblk1 : Inport
  cfblk10 : Inport  Port=2
  cfblk11 : Inport  Port=3
  cfblk12 : Inport  Port=4
  cfblk13 : Inport  Port=5
  cfblk14 : Inport  Port=6
  cfblk15 : Inport  Port=7
  cfblk3 : MinMax
  cfblk4 : Reshape
  cfblk5 : simulink/Math Operations/Slider Gain  gain=1  low=0  high=2
  cfblk6 : simulink/Math Operations/MinMax Running Resettable  Function=min  vinit=0.0
  cfblk7 : Sum  Inputs=+
  cfblk8 : Bias  Bias=[-58067725.138450]
  cfblk9 : Product  Inputs=**
  cfblk2 : Outport
  cfblk16 : Outport  Port=2
  cfblk17 : Outport  Port=3
  wires:
  cfblk8/1 -> cfblk9/1
  cfblk14/1 -> cfblk7/1
  cfblk5/1 -> cfblk6/1
  cfblk10/1 -> cfblk2/1
  cfblk11/1 -> cfblk4/1
  cfblk4/1 -> cfblk3/1
  cfblk3/1 -> cfblk16/1
  cfblk13/1 -> cfblk6/2
  cfblk7/1 -> cfblk8/1
  cfblk1/1 -> cfblk17/1
  cfblk12/1 -> cfblk5/1
  cfblk6/1 -> cfblk9/2

== system sampleModel20/cfblk94/cfblk11/cfblk6/cfblk4 ==
  cfblk1 : Inport
  cfblk9 : Inport  Port=2
  cfblk10 : Inport  Port=3
  cfblk11 : Inport  Port=4
  cfblk12 : Inport  Port=5
  cfblk13 : Inport  Port=6
  cfblk18 : Delay  SampleTime=1
  cfblk3 : UnaryMinus
  cfblk4 : Sum
  cfblk5 : Product  Inputs=**
  cfblk6 : Product  Inputs=**
  cfblk7 : PermuteDimensions
  cfblk8 : Math  Operator=conj  SaturateOnIntegerOverflow=on
  cfblk2 : Outport
  cfblk14 : Outport  Port=2
  cfblk15 : Outport  Port=3
  cfblk16 : Outport  Port=4
  cfblk17 : Outport  Port=5
  wires:
  cfblk7/1 -> cfblk15/1, cfblk14/1
  cfblk6/1 -> cfblk3/1, cfblk5/2
  cfblk11/1 -> cfblk2/1
  cfblk1/1 -> cfblk6/2
  cfblk8/1 -> cfblk4/1
  cfblk12/1 -> cfblk8/1
  cfblk3/1 -> cfblk4/2
  cfblk13/1 -> cfblk7/1
  cfblk10/1 -> cfblk5/1
  cfblk5/1 -> cfblk16/1
  cfblk9/1 -> cfblk17/1
  cfblk4/1 -> cfblk18/1
  cfblk18/1 -> cfblk6/1

== system sampleModel20/cfblk94/cfblk11/cfblk6/cfblk5 ==
  cfblk1 : Inport
  cfblk4 : Inport  Port=2
  cfblk5 : Inport  Port=3
  cfblk6 : Inport  Port=4
  cfblk3 : pid_lib/PID Controller (2DOF)  Controller=PID  Form=Parallel  TimeDomain=Discrete-time  UseExternalTs=off  SampleTime=1  IntegratorMethod=Forward Euler  FilterMethod=Forward Euler  ControllerParametersSource=internal  P=1  I=1  D=0  UseFilter=on  N=100  b=1  c=1  TunerSelectOption=Transfer Function Based (PID Tuner App)  InitialConditionSource=internal  InitialConditionForIntegrator=0  InitialConditionForFilter=0  DifferentiatorICPrevScaledInput=0  ExternalReset=none  TrackingMode=off  Kt=1  LimitOutput=off  SatLimitsSource=internal  UpperSaturationLimit=inf  LowerSaturationLimit=-inf  LinearizeAsGain=off  AntiWindupMode=none  Kb=1  POutMin=[]  POutMax=[]  IOutMin=[]  IOutMax=[]  DOutMin=[]  DOutMax=[]  NOutMin=[]  NOutMax=[]  bOutMin=[]  bOutMax=[]  cOutMin=[]  cOutMax=[]  SumOutMin=[]  SumOutMax=[]  SaturationOutMin=[]  SaturationOutMax=[]  PParamMin=[]  PParamMax=[]  IParamMin=[]  IParamMax=[]  DParamMin=[]  DParamMax=[]  NParamMin=[]  NParamMax=[]  bParamMin=[]  bParamMax=[]  cParamMin=[]  cParamMax=[]  KbParamMin=[]  KbParamMax=[]  KtParamMin=[]  KtParamMax=[]  KbOutMin=[]  KbOutMax=[]  KtOutMin=[]  KtOutMax=[]  IntegratorOutMin=[]  IntegratorOutMax=[]  FilterOutMin=[]  FilterOutMax=[]  SumI1OutMin=[]  SumI1OutMax=[]  SumI2OutMin=[]  SumI2OutMax=[]  SumI3OutMin=[]  SumI3OutMax=[]  SumI4OutMin=[]  SumI4OutMax=[]  SumDOutMin=[]  SumDOutMax=[]  Sum1OutMin=[]  Sum1OutMax=[]  Sum2OutMin=[]  Sum2OutMax=[]  Sum3OutMin=[]  Sum3OutMax=[]  DifferentiatorOutMin=[]  DifferentiatorOutMax=[]  FilterDiffOutCoefMin=[]  FilterDiffOutCoefMax=[]  ReciprocalOutMin=[]  ReciprocalOutMax=[]  SumDenOutMin=[]  SumDenOutMax=[]  SumNumOutMin=[]  SumNumOutMax=[]  DivideOutMin=[]  DivideOutMax=[]  UdiffTsProdOutMin=[]  UdiffTsProdOutMax=[]  NTsProdOutMin=[]  NTsProdOutMax=[]  UintegralTsProdOutMin=[]  UintegralTsProdOutMax=[]  UngainTsProdOutMin=[]  UngainTsProdOutMax=[]  IntegratorContinuousStateAttributes=''  IntegratorStateMustResolveToSignalObject=off  IntegratorRTWStateStorageClass=Auto  FilterContinuousStateAttributes=''  FilterStateMustResolveToSignalObject=off  FilterRTWStateStorageClass=Auto  ParallelPVariant=InternalParameters  IdealPVariant=Disabled  IVariant=InternalParameters  DVariant=InternalParameters  bVariant=InternalParameters  cVariant=InternalParameters  IntegratorVariant=Discrete  SatVariant=Disabled  AWVariant=Passthrough  PCopyVariant=Disabled  TRVariant=Disabled  FdbkBlocksVariant=Forward  IdealPFdbkVariant=Disabled  SatFdbkVariant=Disabled  DerivativeFilterVariant=ForwardEulerFilter  NVariant=InternalParameters  NCopyVariant=Disabled  FilterICVariant=InternalICsFilter  IntegratorICVariant=InternalICs  ExternalResetVariant=Disabled  TRSumVariant=Passthrough  SumFdbkVariant=Disabled  SumVariant=Sum_PID  TsampFilterVariant=InternalTs  TsampNgainVariant=Passthrough  TsampIntegralVariant=Passthrough  ExternalSaturationOutDataTypeStr=Inherit: Same as second input
      settings: SourceProductBaseCode=SL
  cfblk2 : Outport
  cfblk7 : Outport  Port=2
  cfblk8 : Outport  Port=3
  wires:
  cfblk1/1 -> cfblk3/1
  cfblk5/1 -> cfblk2/1
  cfblk6/1 -> cfblk3/2
  cfblk4/1 -> cfblk8/1
  cfblk3/1 -> cfblk7/1

== system sampleModel20/cfblk94/cfblk11/cfblk7/cfblk4 ==
  cfblk1 : Inport
  cfblk8 : Inport  Port=2
  cfblk9 : Inport  Port=3
  cfblk10 : Inport  Port=4
  cfblk11 : Delay  SampleTime=1
  cfblk3 : Assignment  DiagnosticForDimensions=Warning  IndexOptions=Index vector (dialog)  Indices=1  OutputSizes=1
  cfblk4 : Sqrt  Operator=rSqrt  AlgorithmType=Newton-Raphson  SaturateOnIntegerOverflow=on
  cfblk5 : Product  Inputs=**
  cfblk6 : Squeeze
  cfblk7 : simulink/Math Operations/MinMax Running Resettable  Function=min  vinit=0.0
  cfblk2 : Outport
  wires:
  cfblk7/1 -> cfblk5/1
  cfblk10/1 -> cfblk4/1
  cfblk8/1 -> cfblk2/1
  cfblk9/1 -> cfblk5/2
  cfblk1/1 -> cfblk7/2
  cfblk5/1 -> cfblk6/1
  cfblk6/1 -> cfblk3/1
  cfblk4/1 -> cfblk3/2
  cfblk3/1 -> cfblk11/1
  cfblk11/1 -> cfblk7/1

== system sampleModel20/cfblk94/cfblk11/cfblk7/cfblk5 ==
  cfblk1 : Inport
  cfblk9 : Inport  Port=2
  cfblk10 : Inport  Port=3
  cfblk11 : Inport  Port=4
  cfblk3 : UnaryMinus
  cfblk4 : UnaryMinus
  cfblk5 : simulink/Math Operations/MinMax Running Resettable  Function=min  vinit=0.0
  cfblk6 : ComplexToMagnitudeAngle
  cfblk7 : Product
  cfblk8 : Sum  Inputs=|++
  cfblk2 : Outport
  wires:
  cfblk3/1 -> cfblk5/1
  cfblk10/1 -> cfblk7/1
  cfblk7/1 -> cfblk5/2
  cfblk1/1 -> cfblk2/1
  cfblk9/1 -> cfblk6/1
  cfblk5/1 -> cfblk8/1
  cfblk6/1 -> cfblk3/1
  cfblk4/1 -> cfblk7/2
  cfblk6/2 -> cfblk4/1
  cfblk11/1 -> cfblk8/2

== system sampleModel20/cfblk94/cfblk6/cfblk7/cfblk5 ==
  cfblk1 : Inport
  cfblk6 : Inport  Port=2
  cfblk7 : Inport  Port=3
  cfblk8 : Inport  Port=4
  cfblk9 : Inport  Port=5
  cfblk10 : Inport  Port=6
  cfblk11 : Inport  Port=7
  cfblk12 : Delay  SampleTime=1
  cfblk3 : Assignment  DiagnosticForDimensions=Warning  IndexOptions=Index vector (dialog)  Indices=1  OutputSizes=1
  cfblk4 : Polyval  Coefs=[ +2.081618890e-019, -1.441693666e-014, +4.719686976e-010, -8.536869453e-006, +1.621573104e-001, -8.087801117e+001 ]
  cfblk5 : Gain  Gain=[-558274895.878838]
  cfblk2 : Outport
  wires:
  cfblk4/1 -> cfblk5/1
  cfblk9/1 -> cfblk2/1
  cfblk10/1 -> cfblk3/1
  cfblk3/1 -> cfblk4/1
  cfblk5/1 -> cfblk12/1
  cfblk12/1 -> cfblk3/2

== system sampleModel20/cfblk94/cfblk6/cfblk7/cfblk6 ==
  cfblk1 : Inport
  cfblk8 : Inport  Port=2
  cfblk9 : Inport  Port=3
  cfblk10 : Inport  Port=4
  cfblk11 : Inport  Port=5
  cfblk12 : Inport  Port=6
  cfblk13 : Inport  Port=7
  cfblk14 : Inport  Port=8
  cfblk3 : Sqrt  SaturateOnIntegerOverflow=on
  cfblk4 : Sum  Inputs=+
  cfblk5 : Trigonometry
  cfblk6 : UnaryMinus
  cfblk7 : Rounding
  cfblk2 : Outport
  cfblk15 : Outport  Port=2
  wires:
  cfblk4/1 -> cfblk3/1
  cfblk6/1 -> cfblk4/1
  cfblk12/1 -> cfblk6/1
  cfblk10/1 -> cfblk2/1
  cfblk14/1 -> cfblk7/1
  cfblk5/1 -> cfblk15/1
  cfblk3/1 -> cfblk5/1

== system sampleModel20/cfblk94/cfblk6/cfblk7/cfblk7 ==
  cfblk1 : Inport
  cfblk10 : Inport  Port=2
  cfblk11 : Inport  Port=3
  cfblk12 : Inport  Port=4
  cfblk13 : Inport  Port=5
  cfblk14 : Inport  Port=6
  cfblk15 : Inport  Port=7
  cfblk16 : Inport  Port=8
  cfblk18 : Delay  SampleTime=1
  cfblk3 : Math  Operator=10^u  SaturateOnIntegerOverflow=on
  cfblk4 : Sum  Inputs=+
  cfblk5 : UnaryMinus
  cfblk6 : simulink/Math Operations/MinMax Running Resettable  Function=min  vinit=0.0
  cfblk7 : DotProduct  InputSameDT=on  OutDataTypeStr=Inherit: Inherit via internal rule
  cfblk8 : Sqrt  SaturateOnIntegerOverflow=on
  cfblk9 : simulink/Math Operations/Slider Gain  gain=1  low=0  high=2
  cfblk2 : Outport
  cfblk17 : Outport  Port=2
  wires:
  cfblk9/1 -> cfblk5/1
  cfblk14/1 -> cfblk3/1
  cfblk7/1 -> cfblk8/1
  cfblk1/1 -> cfblk4/1
  cfblk16/1 -> cfblk2/1
  cfblk13/1 -> cfblk9/1
  cfblk10/1 -> cfblk17/1
  cfblk5/1 -> cfblk7/1
  cfblk15/1 -> cfblk6/1
  cfblk4/1 -> cfblk6/2
  cfblk8/1 -> cfblk18/1
  cfblk18/1 -> cfblk7/2

== system sampleModel20/cfblk94/cfblk6/cfblk7/cfblk8 ==
  cfblk1 : Inport
  cfblk7 : Inport  Port=2
  cfblk8 : Inport  Port=3
  cfblk9 : Inport  Port=4
  cfblk10 : Inport  Port=5
  cfblk11 : Inport  Port=6
  cfblk12 : Inport  Port=7
  cfblk13 : Inport  Port=8
  cfblk16 : Delay  SampleTime=1
  cfblk3 : Assignment  DiagnosticForDimensions=Warning  IndexOptions=Index vector (dialog)  Indices=1  OutputSizes=1
  cfblk4 : Sqrt  SaturateOnIntegerOverflow=on
  cfblk5 : Product
  cfblk6 : Abs
  cfblk2 : Outport
  cfblk14 : Outport  Port=2
  cfblk15 : Outport  Port=3
  wires:
  cfblk12/1 -> cfblk2/1
  cfblk10/1 -> cfblk15/1
  cfblk3/1 -> cfblk6/1
  cfblk7/1 -> cfblk3/1
  cfblk6/1 -> cfblk14/1
  cfblk5/1 -> cfblk4/1
  cfblk9/1 -> cfblk3/2
  cfblk1/1 -> cfblk5/2
  cfblk4/1 -> cfblk16/1
  cfblk16/1 -> cfblk5/1

== system sampleModel20/cfblk94/cfblk6/cfblk8/cfblk5 ==
  cfblk1 : Inport
  cfblk9 : Inport  Port=2
  cfblk10 : Inport  Port=3
  cfblk11 : Inport  Port=4
  cfblk12 : Inport  Port=5
  cfblk13 : Inport  Port=6
  cfblk14 : Inport  Port=7
  cfblk15 : Inport  Port=8
  cfblk3 : Polyval  Coefs=[ +2.081618890e-019, -1.441693666e-014, +4.719686976e-010, -8.536869453e-006, +1.621573104e-001, -8.087801117e+001 ]
  cfblk4 : simulink/Math Operations/MinMax Running Resettable  Function=min  vinit=0.0
  cfblk5 : Squeeze
  cfblk6 : Sqrt  Operator=rSqrt  AlgorithmType=Newton-Raphson  SaturateOnIntegerOverflow=on
  cfblk7 : Sum  Inputs=--
  cfblk8 : Product  Inputs=*
  cfblk2 : Outport
  cfblk16 : Outport  Port=2
  wires:
  cfblk14/1 -> cfblk3/1
  cfblk3/1 -> cfblk5/1
  cfblk5/1 -> cfblk8/1
  cfblk1/1 -> cfblk4/1
  cfblk4/1 -> cfblk16/1
  cfblk6/1 -> cfblk2/1
  cfblk12/1 -> cfblk7/1
  cfblk15/1 -> cfblk6/1
  cfblk11/1 -> cfblk4/2
  cfblk9/1 -> cfblk7/2

== system sampleModel20/cfblk94/cfblk6/cfblk8/cfblk6 ==
  cfblk1 : Inport
  cfblk9 : Inport  Port=2
  cfblk10 : Inport  Port=3
  cfblk11 : Inport  Port=4
  cfblk12 : Inport  Port=5
  cfblk13 : Inport  Port=6
  cfblk14 : Inport  Port=7
  cfblk16 : Delay  SampleTime=1
  cfblk3 : pid_lib/PID Controller  Controller=PID  Form=Parallel  TimeDomain=Discrete-time  UseExternalTs=off  SampleTime=1  IntegratorMethod=Forward Euler  FilterMethod=Forward Euler  ControllerParametersSource=internal  P=1  I=1  D=0  UseFilter=on  N=100  TunerSelectOption=Transfer Function Based (PID Tuner App)  InitialConditionSource=internal  InitialConditionForIntegrator=0  InitialConditionForFilter=0  DifferentiatorICPrevScaledInput=0  ExternalReset=none  TrackingMode=off  Kt=1  LimitOutput=off  SatLimitsSource=internal  UpperSaturationLimit=inf  LowerSaturationLimit=-inf  LinearizeAsGain=off  AntiWindupMode=none  Kb=1  POutMin=[]  POutMax=[]  IOutMin=[]  IOutMax=[]  DOutMin=[]  DOutMax=[]  NOutMin=[]  NOutMax=[]  SumOutMin=[]  SumOutMax=[]  SaturationOutMin=[]  SaturationOutMax=[]  PParamMin=[]  PParamMax=[]  IParamMin=[]  IParamMax=[]  DParamMin=[]  DParamMax=[]  NParamMin=[]  NParamMax=[]  KbParamMin=[]  KbParamMax=[]  KtParamMin=[]  KtParamMax=[]  KbOutMin=[]  KbOutMax=[]  KtOutMin=[]  KtOutMax=[]  IntegratorOutMin=[]  IntegratorOutMax=[]  FilterOutMin=[]  FilterOutMax=[]  SumI1OutMin=[]  SumI1OutMax=[]  SumI2OutMin=[]  SumI2OutMax=[]  SumI3OutMin=[]  SumI3OutMax=[]  SumI4OutMin=[]  SumI4OutMax=[]  SumDOutMin=[]  SumDOutMax=[]  DifferentiatorOutMin=[]  DifferentiatorOutMax=[]  FilterDiffOutCoefMin=[]  FilterDiffOutCoefMax=[]  ReciprocalOutMin=[]  ReciprocalOutMax=[]  SumDenOutMin=[]  SumDenOutMax=[]  SumNumOutMin=[]  SumNumOutMax=[]  DivideOutMin=[]  DivideOutMax=[]  UdiffTsProdOutMin=[]  UdiffTsProdOutMax=[]  NTsProdOutMin=[]  NTsProdOutMax=[]  UintegralTsProdOutMin=[]  UintegralTsProdOutMax=[]  UngainTsProdOutMin=[]  UngainTsProdOutMax=[]  IntegratorContinuousStateAttributes=''  IntegratorStateMustResolveToSignalObject=off  IntegratorRTWStateStorageClass=Auto  FilterContinuousStateAttributes=''  FilterStateMustResolveToSignalObject=off  FilterRTWStateStorageClass=Auto  ParallelPVariant=InternalParameters  IdealPVariant=Disabled  IVariant=InternalParameters  DVariant=InternalParameters  IntegratorVariant=Discrete  SatVariant=Disabled  AWVariant=Passthrough  PCopyVariant=Disabled  TRVariant=Disabled  FdbkBlocksVariant=Forward  IdealPFdbkVariant=Disabled  SatFdbkVariant=Disabled  DerivativeFilterVariant=ForwardEulerFilter  NVariant=InternalParameters  NCopyVariant=Disabled  FilterICVariant=InternalICsFilter  IntegratorICVariant=InternalICs  ExternalResetVariant=Disabled  TRSumVariant=Passthrough  SumFdbkVariant=Disabled  SumVariant=Sum_PID  TsampFilterVariant=InternalTs  TsampNgainVariant=Passthrough  TsampIntegralVariant=Passthrough  ExternalSaturationOutDataTypeStr=Inherit: Same as second input
  cfblk4 : ComplexToRealImag
  cfblk5 : Squeeze
  cfblk6 : DotProduct  InputSameDT=on  OutDataTypeStr=Inherit: Inherit via internal rule
  cfblk7 : simulink/Math Operations/MinMax Running Resettable  Function=min  vinit=0.0
  cfblk8 : DotProduct  InputSameDT=on  OutDataTypeStr=Inherit: Inherit via internal rule
  cfblk2 : Outport
  cfblk15 : Outport  Port=2
  wires:
  cfblk13/1 -> cfblk2/1
  cfblk7/1 -> cfblk4/1
  cfblk3/1 -> cfblk15/1
  cfblk9/1 -> cfblk3/1
  cfblk10/1 -> cfblk8/1
  cfblk6/1 -> cfblk8/2
  cfblk4/1 -> cfblk6/1
  cfblk12/1 -> cfblk5/1
  cfblk5/1 -> cfblk6/2
  cfblk1/1 -> cfblk7/1
  cfblk8/1 -> cfblk16/1
  cfblk16/1 -> cfblk7/2

== system sampleModel20/cfblk94/cfblk6/cfblk8/cfblk7 ==
  cfblk1 : Inport
  cfblk9 : Inport  Port=2
  cfblk10 : Inport  Port=3
  cfblk11 : Inport  Port=4
  cfblk12 : Inport  Port=5
  cfblk13 : Inport  Port=6
  cfblk17 : Delay  SampleTime=1
  cfblk3 : Delay  DelayLengthSource=Input port  SampleTime=1
      settings: InputPortMap=u0,p1
  cfblk4 : Product  Inputs=*
  cfblk5 : Reshape
  cfblk6 : DotProduct  InputSameDT=on  OutDataTypeStr=Inherit: Inherit via internal rule
  cfblk7 : simulink/Math Operations/Slider Gain  gain=1  low=0  high=2
  cfblk8 : UnaryMinus
  cfblk2 : Outport
  cfblk14 : Outport  Port=2
  cfblk15 : Outport  Port=3
  cfblk16 : Outport  Port=4
  wires:
  cfblk5/1 -> cfblk6/1
  cfblk13/1 -> cfblk2/1
  cfblk10/1 -> cfblk16/1
  cfblk8/1 -> cfblk7/1, cfblk4/1
  cfblk12/1 -> cfblk5/1
  cfblk1/1 -> cfblk15/1
  cfblk9/1 -> cfblk3/1
  cfblk6/1 -> cfblk8/1
  cfblk3/1 -> cfblk14/1
  cfblk11/1 -> cfblk3/2
  cfblk7/1 -> cfblk17/1
  cfblk17/1 -> cfblk6/2

== system sampleModel20/cfblk94/cfblk6/cfblk8/cfblk8 ==
  cfblk1 : Inport
  cfblk6 : Inport  Port=2
  cfblk7 : Inport  Port=3
  cfblk8 : Inport  Port=4
  cfblk9 : Inport  Port=5
  cfblk10 : Inport  Port=6
  cfblk3 : Sum  Inputs=+-
  cfblk4 : UnaryMinus
  cfblk5 : Signum
  cfblk2 : Outport
  cfblk11 : Outport  Port=2
  wires:
  cfblk6/1 -> cfblk2/1
  cfblk5/1 -> cfblk11/1
  cfblk4/1 -> cfblk5/1
  cfblk7/1 -> cfblk4/1
  cfblk10/1 -> cfblk3/1
  cfblk8/1 -> cfblk3/2

== system sampleModel20/cfblk94/cfblk7/cfblk4/cfblk5 ==
  cfblk1 : Inport
  cfblk7 : Inport  Port=2
  cfblk3 : Product
  cfblk4 : Trigonometry
  cfblk5 : Bias  Bias=[272949520.451675]
  cfblk6 : Polyval  Coefs=[ +2.081618890e-019, -1.441693666e-014, +4.719686976e-010, -8.536869453e-006, +1.621573104e-001, -8.087801117e+001 ]
  cfblk2 : Outport
  cfblk8 : Outport  Port=2
  wires:
  cfblk7/1 -> cfblk6/1
  cfblk1/1 -> cfblk3/1
  cfblk6/1 -> cfblk3/2
  cfblk3/1 -> cfblk5/1, cfblk4/1
  cfblk5/1 -> cfblk8/1
  cfblk4/1 -> cfblk2/1

== system sampleModel20/cfblk94/cfblk7/cfblk4/cfblk6 ==
  cfblk1 : Inport
  cfblk11 : Inport  Port=2
  cfblk12 : Inport  Port=3
  cfblk13 : Inport  Port=4
  cfblk14 : Inport  Port=5
  cfblk15 : Inport  Port=6
  cfblk16 : Inport  Port=7
  cfblk10 : Sqrt  Operator=rSqrt  AlgorithmType=Newton-Raphson  SaturateOnIntegerOverflow=on
  cfblk3 : Polyval  Coefs=[ +2.081618890e-019, -1.441693666e-014, +4.719686976e-010, -8.536869453e-006, +1.621573104e-001, -8.087801117e+001 ]
  cfblk4 : Sum  Inputs=--
  cfblk5 : Reshape
  cfblk6 : Product  Inputs=**
  cfblk7 : Product
  cfblk8 : Sum  Inputs=+-
  cfblk9 : Reshape
  cfblk2 : Outport
  cfblk17 : Outport  Port=2
  wires:
  cfblk8/1 -> cfblk5/1
  cfblk5/1 -> cfblk17/1
  cfblk6/1 -> cfblk7/1
  cfblk10/1 -> cfblk3/1
  cfblk12/1 -> cfblk7/2
  cfblk7/1 -> cfblk2/1
  cfblk16/1 -> cfblk6/1
  cfblk15/1 -> cfblk9/1
  cfblk3/1 -> cfblk4/1
  cfblk1/1 -> cfblk8/1
  cfblk4/1 -> cfblk8/2
  cfblk13/1 -> cfblk6/2
  cfblk9/1 -> cfblk10/1
  cfblk14/1 -> cfblk4/2

== system sampleModel20/cfblk94/cfblk7/cfblk4/cfblk7 ==
  cfblk1 : Inport
  cfblk7 : Inport  Port=2
  cfblk8 : Inport  Port=3
  cfblk9 : Inport  Port=4
  cfblk12 : Delay  SampleTime=1
  cfblk3 : simulink/Math Operations/MinMax Running Resettable  Function=min  vinit=0.0
  cfblk4 : Squeeze
  cfblk5 : simulink/Math Operations/MinMax Running Resettable  Function=min  vinit=0.0
  cfblk6 : DotProduct  InputSameDT=on  OutDataTypeStr=Inherit: Inherit via internal rule
  cfblk2 : Outport
  cfblk10 : Outport  Port=2
  cfblk11 : Outport  Port=3
  wires:
  cfblk3/1 -> cfblk6/1, cfblk10/1
  cfblk8/1 -> cfblk2/1
  cfblk5/1 -> cfblk3/1
  cfblk4/1 -> cfblk5/2, cfblk6/2
  cfblk7/1 -> cfblk11/1
  cfblk1/1 -> cfblk4/1
  cfblk9/1 -> cfblk3/2
  cfblk6/1 -> cfblk12/1
  cfblk12/1 -> cfblk5/1

== system sampleModel20/cfblk94/cfblk7/cfblk4/cfblk8 ==
  cfblk1 : Inport
  cfblk4 : Inport  Port=2
  cfblk5 : Inport  Port=3
  cfblk6 : Inport  Port=4
  cfblk7 : Inport  Port=5
  cfblk8 : Inport  Port=6
  cfblk9 : Inport  Port=7
  cfblk10 : Inport  Port=8
  cfblk3 : Sum
  cfblk2 : Outport
  cfblk11 : Outport  Port=2
  cfblk12 : Outport  Port=3
  wires:
  cfblk10/1 -> cfblk12/1
  cfblk9/1 -> cfblk11/1
  cfblk1/1 -> cfblk2/1
  cfblk4/1 -> cfblk3/1
  cfblk5/1 -> cfblk3/2

== system sampleModel20/cfblk94/cfblk7/cfblk4/cfblk9 ==
  cfblk1 : Inport
  cfblk8 : Inport  Port=2
  cfblk9 : Inport  Port=3
  cfblk10 : Delay  SampleTime=1
  cfblk3 : MinMax  Function=max  Inputs=3
  cfblk4 : ComplexToMagnitudeAngle
  cfblk5 : Product  Inputs=*
  cfblk6 : Math  Operator=log  SaturateOnIntegerOverflow=on
  cfblk7 : simulink/Math Operations/MinMax Running Resettable  Function=min  vinit=0.0
  cfblk2 : Outport
  wires:
  cfblk4/1 -> cfblk3/1
  cfblk1/1 -> cfblk2/1
  cfblk9/1 -> cfblk3/2
  cfblk4/2 -> cfblk6/1, cfblk7/2
  cfblk8/1 -> cfblk5/1
  cfblk5/1 -> cfblk3/3
  cfblk3/1 -> cfblk7/1
  cfblk6/1 -> cfblk10/1
  cfblk10/1 -> cfblk4/1

== system sampleModel20/cfblk94/cfblk8/cfblk8/cfblk6 ==
  cfblk1 : Inport
  cfblk11 : Inport  Port=2
  cfblk12 : Inport  Port=3
  cfblk10 : Sum  Inputs=+-
  cfblk13 : Delay  SampleTime=1
  cfblk14 : Delay  SampleTime=1
  cfblk3 : Rounding
  cfblk4 : MinMax  Inputs=3
  cfblk5 : PermuteDimensions
  cfblk6 : simulink/Math Operations/Slider Gain  gain=1  low=0  high=2
  cfblk7 : Bias  Bias=[633068473.448704]
  cfblk8 : simulink/Math Operations/MinMax Running Resettable  Function=min  vinit=0.0
  cfblk9 : Polyval  Coefs=[ +2.081618890e-019, -1.441693666e-014, +4.719686976e-010, -8.536869453e-006, +1.621573104e-001, -8.087801117e+001 ]
  cfblk2 : Outport
  wires:
  cfblk10/1 -> cfblk3/1
  cfblk3/1 -> cfblk2/1, cfblk13/1
  cfblk6/1 -> cfblk9/1, cfblk14/1
  cfblk4/1 -> cfblk10/1
  cfblk5/1 -> cfblk7/1
  cfblk1/1 -> cfblk8/1
  cfblk12/1 -> cfblk10/2
  cfblk7/1 -> cfblk6/1
  cfblk9/1 -> cfblk8/2
  cfblk8/1 -> cfblk4/1
  cfblk11/1 -> cfblk4/2
  cfblk13/1 -> cfblk4/3
  cfblk14/1 -> cfblk5/1

== system sampleModel20/cfblk94/cfblk8/cfblk8/cfblk7 ==
  cfblk1 : Inport
  cfblk7 : Inport  Port=2
  cfblk8 : Inport  Port=3
  cfblk9 : Inport  Port=4
  cfblk10 : Inport  Port=5
  cfblk11 : Inport  Port=6
  cfblk12 : Inport  Port=7
  cfblk3 : ComplexToRealImag
  cfblk4 : Sin  TimeSource=Use external signal  SampleTime=0
  cfblk5 : Assignment  DiagnosticForDimensions=Warning  IndexOptions=Index vector (dialog)  Indices=1  OutputSizes=1
  cfblk6 : Bias  Bias=[-573128610.715353]
  cfblk2 : Outport
  wires:
  cfblk7/1 -> cfblk4/1
  cfblk11/1 -> cfblk2/1
  cfblk12/1 -> cfblk6/1
  cfblk9/1 -> cfblk5/1
  cfblk1/1 -> cfblk3/1
  cfblk3/1 -> cfblk5/2
